simulink model "initial_states"  (R2024a)
settings: Solver=FixedStepAuto  StartTime=0.0  StopTime=1  FixedStep=0.5  RelTol=1e-3
settings Model: Creator=jagmohan  LastModifiedBy=jagmohan

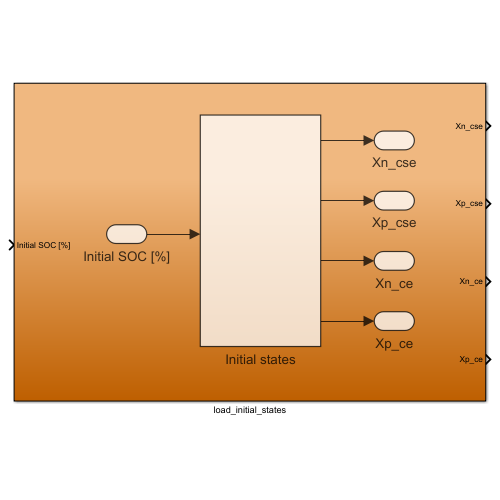
[thumbnail: Simulink's stored preview of the top-level diagram]
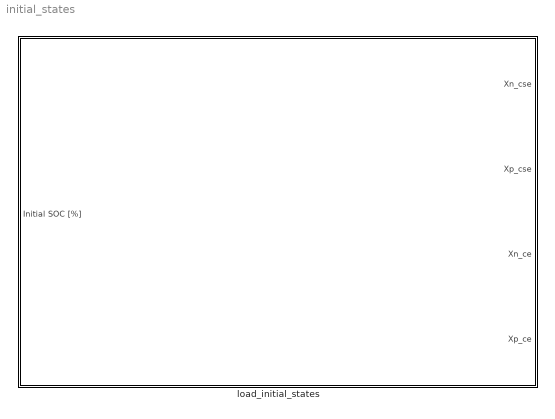
== system initial_states ==
  load_initial_states : Subsystem

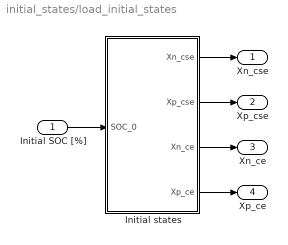
== system initial_states/load_initial_states ==
  Initial SOC [%] : Inport
  Initial states : MATLAB Function  TreatAsAtomicUnit=on
  Xn_cse : Outport
  Xp_cse : Outport  Port=2
  Xn_ce : Outport  Port=3
  Xp_ce : Outport  Port=4
  wires:
  Initial states/4(Xp_ce) -> Xp_ce/1
  Initial states/3(Xn_ce) -> Xn_ce/1
  Initial states/2(Xp_cse) -> Xp_cse/1
  Initial states/1(Xn_cse) -> Xn_cse/1
  Initial SOC [%]/1 -> Initial states/1(SOC_0)

== matlab function initial_states/load_initial_states/Initial states ==
  data: SOC_0 input size=1; Xn_cse output size=3; Xp_cse output size=3; Xn_ce output size=1; Xp_ce output size=1
function [Xn_cse, Xp_cse, Xn_ce, Xp_ce] = fcn(SOC_0)

    
    % Convert SOC from percentage to fraction
    SOC_0 = SOC_0/100;

    %% Fixed parameters
    
    % Limits
    cse_n_max = 33133; % [mol/m^3] max concentration in negative electrode
    cse_p_max = 63104; % [mol/m^3] max concentration in positive electrode
    %Note: Need to update all theta parameters based on the cell
    theta_n_0 = 0.0282; % [-] negative electrode surface stoichiometry when SOC = 0
    theta_n_1 = 0.9014; % [-] negative electrode surface stoichiometry when SOC = 1
    theta_p_0 = 0.9369; % [-] positive electrode surface stoichiometry when SOC = 0
    theta_p_1 = 0.2752; % [-] positive electrode surface stoichiometry when SOC = 1
    
    %% Initialize state-space model
    
    theta_n = (theta_n_1-theta_n_0)*SOC_0+theta_n_0; % [-] initial negative electrode surface stoichiometry
    theta_p = theta_p_0-(theta_p_0-theta_p_1)*SOC_0; % [-] initial positive electrode surface stoichiometry
    cse_0_n = theta_n*cse_n_max; % [mol/m^3] initial concentration of ions in negative solid electrode
    cse_0_p = theta_p*cse_p_max; % [mol/m^3] initial concentration of ions in positive solid electrode

    cse_n_init = zeros(3,1); 
    cse_n_init(1) = cse_0_n/(-1638.19008596954);
    cse_p_init = zeros(3,1); 
    cse_p_init(1) = cse_0_p/(-42.9133048003876);
    ce_n_init = 0;   % IC for electrolyte at n-electrode
    ce_p_init = 0;   % IC for electrolyte at p-electrode

    %%% Initial conditions
    % n-electrode
    Xn_cse = cse_n_init;      
    % p-electrode 
    Xp_cse = cse_p_init;
    % n-lectrolyte
    Xn_ce = ce_n_init;
    % p-electrolyte
    Xp_ce = ce_p_init;

end
